simulink model "permisousuario"  (R2020b)
settings: Solver=VariableStepAuto  StartTime=0.0  StopTime=10.0  RelTol=1e-3
settings Model: Creator=cacha  LastModifiedBy=cacha

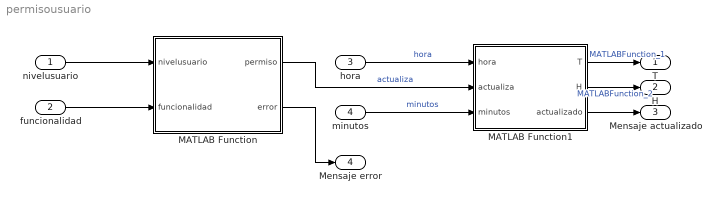
== system permisousuario ==
  nivelusuario : Inport
  funcionalidad : Inport  Port=2
  "hora " : Inport  Port=3  OutMin=0  OutMax=72  OutDataTypeStr=double  PortDimensions=1
  minutos : Inport  Port=4  OutMin=0  OutMax=30  OutDataTypeStr=double  PortDimensions=1
  MATLAB Function : MATLAB Function  TreatAsAtomicUnit=on
  MATLAB Function1 : MATLAB Function  TreatAsAtomicUnit=on
  T : Outport  SignalName=T  OutMin=0  OutMax=35  OutDataTypeStr=double  PortDimensions=1
      settings: MustResolveToSignalObject=on
  H : Outport  Port=2  SignalName=H  OutMin=0  OutMax=1  OutDataTypeStr=double  PortDimensions=1
      settings: MustResolveToSignalObject=on
  Mensaje actualizado : Outport  Port=3  SignalName=actualizado  OutMin=0  OutMax=1  OutDataTypeStr=double  PortDimensions=1
      settings: MustResolveToSignalObject=on
  Mensaje error : Outport  Port=4  SignalName=H  OutMin=0  OutMax=1  OutDataTypeStr=double  PortDimensions=1
      settings: MustResolveToSignalObject=on
  wires:
  funcionalidad/1 -> MATLAB Function/2(funcionalidad)
  nivelusuario/1 -> MATLAB Function/1(nivelusuario)
  "hora "/1 -> MATLAB Function1/1(hora)  "hora"
  MATLAB Function1/3(actualizado) -> Mensaje actualizado/1
  minutos/1 -> MATLAB Function1/3(minutos)  "minutos"
  MATLAB Function1/2(H) -> H/1  "MATLABFunction_2"
  MATLAB Function/1(permiso) -> MATLAB Function1/2(actualiza)  "actualiza"
  MATLAB Function1/1(T) -> T/1  "MATLABFunction_1"
  MATLAB Function/2(error) -> Mensaje error/1

== matlab function permisousuario/MATLAB Function1 ==
  data: hora input; T output; actualiza input; H output; minutos input; actualizado output
function [T,H,actualizado] = fcn(hora,actualiza,minutos)

persistent x0 

if hora==24 || actualiza == 1 || minutos == 30
%significará que ha pasado de día o cada 
%media hora, o se ha pedido actualizar por el usuario

if isempty(x0)
   x0=1651255;
end
m=2^31;
x0=rem(314159269*x0+453806245,m);
uniforme=x0/m;

    T = uniforme * 35;
    disp('La temperatura de hoy es de');
%     disp(T);

    H = uniforme;
    disp('La humedad de hoy es de');
%     disp(H);
    
    T1 = uniforme * 35;
    disp('La temperatura de mañana es de');
    disp(T1);

    H1 = uniforme;
    disp('La humedad de mañana es de');
    disp(H1);
    
    T2 = uniforme * 35;
    disp('La temperatura de pasado mañana es de');
    disp(T2);

    H2 = uniforme;
    disp('La humedad de pasado mañana es de');
    disp(H2);  
    hora = 0;
    actualizado = 1;
else 
    T = 0;
    H = 0;
    actualizado = 0;
end

end

== matlab function permisousuario/MATLAB Function ==
  data: nivelusuario input; permiso output; funcionalidad input; error output
function [permiso,error] = fcn(nivelusuario, funcionalidad)

if nivelusuario == 1 && (funcionalidad == 1 || funcionalidad == 2 || funcionalidad ==3)
    permiso = 1;
    error = 0;   
elseif nivelusuario == 2 && (funcionalidad == 2 || funcionalidad ==3)
    permiso = 1;
    error = 0;    
elseif nivelusuario ==3 && funcionalidad == 3
    permiso = 1;
    error = 0;

else 
    permiso = 0;
    error = 0;
end

if nivelusuario > funcionalidad 
    error = 1;
end

end
